simulink model "RL_RefAdjSup"  (R2025b)
settings: Solver=ode14x  StartTime=0.0  StopTime=10.0  FixedStep=Ts_local  RelTol=1e-3
model workspace (MAT data in the model file):
  FSI_max = [111.58614649; 109.244229433; 111.951462771]
  FSI_min = [3.65502707696; 3.64264743495; 3.42913459589]
  K1 = 1
  K2 = 1e-06
  Ncycle = 25
  SampEn_max = [0.399850516102; 0.373441099122; 0.45958437331]
  SampEn_min = [0.118794892672; 0.117721768048; 0.119599512992]
  fs = 5000
  m = 2
  rRatio = 0.2
values from neighbouring files (symbols this model uses):
  f = 50.0    [ctrlSys.sldd]
  Ts_ctrl = 0.1    [ctrlSys.sldd]
  Ts_local = 1.0E-5    [ctrlSys.sldd]
  Ts_meas = 0.005    [ctrlSys.sldd]
libraries: rllib x1
settings Model: DataDictionary=ctrlSys.sldd  Creator=i336  LastModifiedBy=LYG

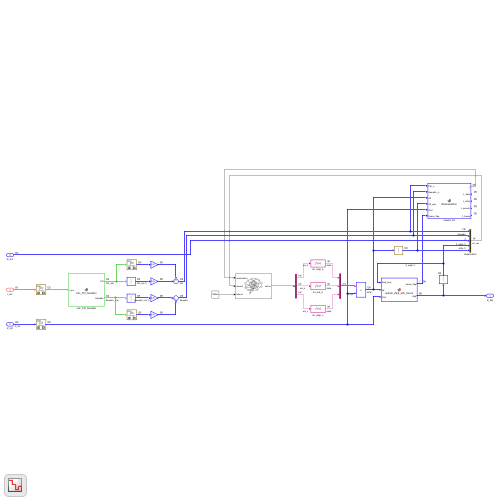
[thumbnail: Simulink's stored preview of the top-level diagram]
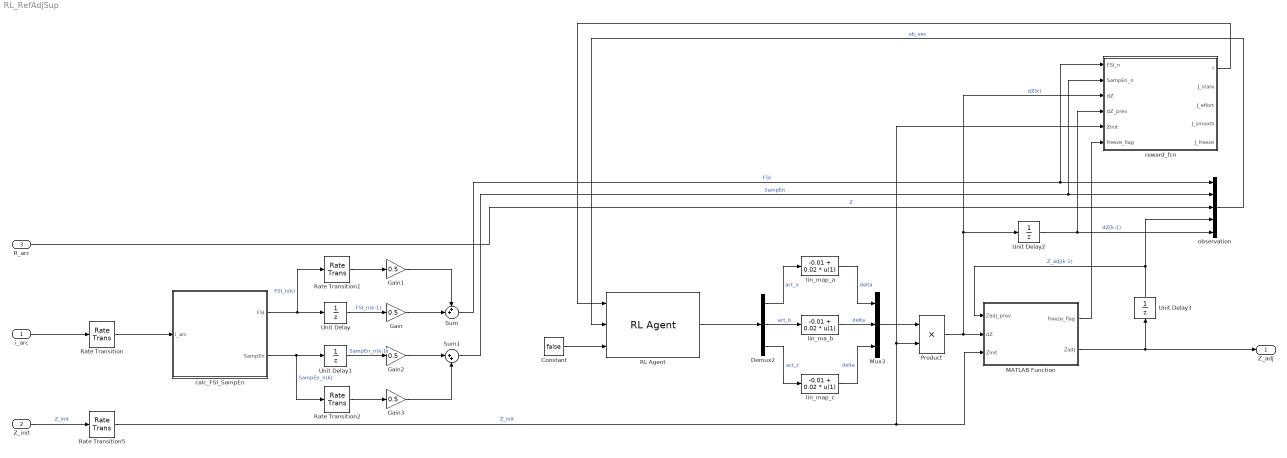
== system RL_RefAdjSup ==
  i_arc : Inport  SampleTime=Ts_local
  Z_init : Inport  Port=2  PortDimensions=[3 1]  SampleTime=Ts_ctrl
  R_arc : Inport  Port=3  PortDimensions=3  SampleTime=Ts_meas
  Constant : Constant  Value=false
  Demux2 : Demux  Outputs=3
  Gain{,1..3} (4 alike) : Gain  Gain=0.5
  MATLAB Function : MATLAB Function  TreatAsAtomicUnit=on
  Mux3 : Mux  Inputs=3
  Product : Product
  RL Agent : rllib/RL Agent  Agent=agentObj  ExternalActionAsInput=off  ProvideLastAction=off  ProvideCumRwd=off  TreatAsDirectFeedthrough=on  UseStrictObservationDataTypes=off
  Rate Transition : RateTransition  OutPortSampleTime=1 / fs
  Rate Transition1 : RateTransition  OutPortSampleTime=Ncycle * (1 / f)
  Rate Transition2 : RateTransition  OutPortSampleTime=Ncycle * (1 / f)
  Rate Transition5 : RateTransition  OutPortSampleTime=Ts_sup
  Sum : Sum  Inputs=++|
  Sum1 : Sum  Inputs=|++
  Unit Delay : UnitDelay  SampleTime=Ncycle * (1 / f)  HasFrameUpgradeWarning=on
  Unit Delay1 : UnitDelay  SampleTime=Ncycle * (1 / f)  HasFrameUpgradeWarning=on
  Unit Delay2 : UnitDelay  SampleTime=-1  HasFrameUpgradeWarning=on
  Unit Delay3 : UnitDelay  SampleTime=-1  HasFrameUpgradeWarning=on
  calc_FSI_SampEn : MATLAB Function  TreatAsAtomicUnit=on  SystemSampleTime=1 / fs
  lin_ma_b : Fcn  Expr=-0.01 + 0.02 * u(1)
  lin_map_a : Fcn  Expr=-0.01 + 0.02 * u(1)
  lin_map_c : Fcn  Expr=-0.01 + 0.02 * u(1)
  observation : Mux  Inputs=5
  reward_fcn : MATLAB Function  TreatAsAtomicUnit=on
  Z_adj : Outport
  wires:
  i_arc/1 -> Rate Transition/1
  Rate Transition/1 -> calc_FSI_SampEn/1(i_arc)
  calc_FSI_SampEn/1(FSI) -> Rate Transition1/1, Unit Delay/1  "FSI_n(k)"
  calc_FSI_SampEn/2(SampEn) -> Rate Transition2/1, Unit Delay1/1  "SampEn_n(k)"
  Unit Delay/1 -> Gain/1  "FSI_n(k-1)"
  Gain/1 -> Sum/2
  Gain1/1 -> Sum/1
  Gain2/1 -> Sum1/1
  Gain3/1 -> Sum1/2
  Unit Delay1/1 -> Gain2/1  "SampEn_n(k-1)"
  Rate Transition1/1 -> Gain1/1
  Rate Transition2/1 -> Gain3/1
  Z_init/1 -> Rate Transition5/1  "Z_init"
  Mux3/1 -> Product/1
  lin_map_a/1 -> Mux3/1  "delta"
  lin_ma_b/1 -> Mux3/2  "delta"
  lin_map_c/1 -> Mux3/3  "delta"
  Sum/1 -> reward_fcn/1(FSI_n), observation/1  "FSI"
  Sum1/1 -> reward_fcn/2(SampEn_n), observation/2  "SampEn"
  Rate Transition5/1 -> MATLAB Function/3(Zinit), Product/2, reward_fcn/5(Zinit)  "Z_init"
  Product/1 -> MATLAB Function/2(dZ), reward_fcn/3(dZ), Unit Delay2/1  "dZ(k)"
  MATLAB Function/2(Zadj) -> Z_adj/1, Unit Delay3/1
  Unit Delay3/1 -> observation/4, MATLAB Function/1(Zadj_prev)  "Z_adj(k-1)"
  R_arc/1 -> observation/3  "Z"
  Unit Delay2/1 -> reward_fcn/4(dZ_prev), observation/5  "dZ(k-1)"
  MATLAB Function/1(freeze_flag) -> reward_fcn/6(freeze_flag)
  Demux2/1 -> lin_map_a/1  "act_a"
  Demux2/2 -> lin_ma_b/1  "act_b"
  Demux2/3 -> lin_map_c/1  "act_c"
  Constant/1 -> RL Agent/3
  RL Agent/1 -> Demux2/1
  observation/1 -> RL Agent/2  "ob_vec"
  reward_fcn/1(r) -> RL Agent/1

== matlab function RL_RefAdjSup/reward_fcn ==
  data: FSI_n input; r output; SampEn_n input; dZ input; dZ_prev input; Zinit input; freeze_flag input; J_state output; J_effort output; J_smooth output; J_freeze output
function [r, J_state, J_effort, J_smooth, J_freeze] = RLRewardFcn( ...
    FSI_n, SampEn_n, dZ, dZ_prev, Zinit, freeze_flag)
%#codegen
% RL reward for variable-impedance supervisory control
%
% Inputs:
%   FSI_n       : 3x1 normalized FSI in [0,1]
%   SampEn_n    : 3x1 normalized SampEn in [0,1]
%   dZ          : 3x1 current impedance increment (physical value)
%   dZ_prev     : 3x1 previous impedance increment (physical value)
%   Zinit       : 3x1 initial/base impedance
%   freeze_flag : 3x1, 1 if corresponding phase update is frozen, else 0
%
% Outputs:
%   r           : scalar reward
%   J_state     : state-quality cost
%   J_effort    : control-effort cost
%   J_smooth    : smoothness cost
%   J_freeze    : freeze penalty cost

    % ---------- Hard-coded weights ----------
    alphaF = 1.0;   % weight of FSI term inside state cost
    alphaS = 1.0;   % weight of SampEn term inside state cost

    beta1  = 0.10;  % weight of effort penalty
    beta2  = 0.20;  % weight of smoothness penalty
    beta3  = 0.50;  % weight of freeze penalty
    % ----------------------------------------

    % Ensure column vectors
    FSI_n       = FSI_n(:);
    SampEn_n    = SampEn_n(:);
    dZ          = dZ(:);
    dZ_prev     = dZ_prev(:);
    Zinit       = Zinit(:);
    freeze_flag = freeze_flag(:);

    % Clamp normalized features to [0,1] for safety
    FSI_n    = min(max(FSI_n, 0.0), 1.0);
    SampEn_n = min(max(SampEn_n, 0.0), 1.0);

    % Convert physical dZ to normalized action-like variable in [-1,1]
    %
    % Forward mapping used previously:
    %   dZ = Zinit * (-0.01 + 0.02 * a),   a in [-1,1]
    %
    % Inverse mapping:
    %   a = (dZ./Zinit + 0.01) / 0.02
    %
    % This normalization makes the effort/smoothness terms dimensionless.
    eps_z = 1e-9;
    Zsafe = max(abs(Zinit), eps_z);

    dZ_n      = (dZ      ./ Zsafe + 0.01) / 0.02;
    dZ_prev_n = (dZ_prev ./ Zsafe + 0.01) / 0.02;

    % Optional clamping for robustness
    dZ_n      = min(max(dZ_n,      -1.0), 1.0);
    dZ_prev_n = min(max(dZ_prev_n, -1.0), 1.0);

    % 1) Buried-arc state cost
    % Larger FSI is better, smaller SampEn is better
    J_state = sum(alphaF * (1.0 - FSI_n) + alphaS * SampEn_n);

    % 2) Control-effort cost
    J_effort = sum(dZ_n.^2);

    % 3) Smoothness cost
    J_smooth = sum((dZ_n - dZ_prev_n).^2);

    % 4) Freeze penalty
    J_freeze = sum(freeze_flag ~= 0);

    % Final reward
    r = -J_state ...
        - beta1 * J_effort ...
        - beta2 * J_smooth ...
        - beta3 * J_freeze;
end

== matlab function RL_RefAdjSup/calc_FSI_SampEn ==
  data: i_arc input size=[3 1]; FSI output; SampEn output; K1 parameter size=[1 1]; K2 parameter size=[1 1]; fs parameter size=[1 1]; Ncycle parameter size=[1 1]; f parameter size=[1 1]; m parameter size=[1 1]; rRatio parameter size=[1 1]; FSI_max parameter size=[3 1]; FSI_min parameter size=[3 1]; SampEn_max parameter size=[3 1]; SampEn_min parameter size=[3 1]
function [FSI, SampEn] = calc_FSI_SampEn( ...
    i_arc, K1, K2, fs, Ncycle, f, m, rRatio, ...
    FSI_max, FSI_min, SampEn_max, SampEn_min)
%#codegen
% i_arc   : 3x1 instantaneous arc current [ia; ib; ic]
% FSI     : 3x1 normalized FSI of three phases
% SampEn  : 3x1 normalized sample entropy of three phases
%
% This version:
% 1) stores samples every call,
% 2) computes features only once every Nhop samples,
% 3) holds the last computed outputs between updates.

    Nwin = int32(Ncycle * fs / f);   % assume exact integer
    Nhop = Nwin;                     % non-overlapping windows
    % For overlapped windows, e.g.:
    % Nhop = int32(Nwin/2);

    persistent buf head count sinceCalc lastFSI lastSampEn

    if isempty(head)
        buf        = zeros(Nwin, 3);
        head       = int32(0);
        count      = int32(0);
        sinceCalc  = int32(0);
        lastFSI    = zeros(3,1);
        lastSampEn = zeros(3,1);
    end

    % Ensure column vector
    i_arc = reshape(i_arc, 3, 1);

    % -------------------------
    % 1) Update circular buffer
    % -------------------------
    head = head + 1;
    if head > Nwin
        head = int32(1);
    end

    buf(head, :) = i_arc.';

    if count < Nwin
        count = count + 1;
    end

    sinceCalc = sinceCalc + 1;

    % Default outputs: hold last values
    FSI    = lastFSI;
    SampEn = lastSampEn;

    % Before first full window, output zeros
    if count < Nwin
        FSI(:)    = 0.0;
        SampEn(:) = 0.0;
        return;
    end

    % -----------------------------------------
    % 2) Only recompute once every Nhop samples
    % -----------------------------------------
    if sinceCalc < Nhop
        return;
    end
    sinceCalc = int32(0);

    % Reconstruct ordered window: oldest --> newest
    xwin = zeros(Nwin, 3);
    if head < Nwin
        n1 = Nwin - head;
        xwin(1:n1, :)      = buf(head+1:Nwin, :);
        xwin(n1+1:Nwin, :) = buf(1:head, :);
    else
        xwin = buf;
    end

    % Compute features phase by phase
    for p = 1:3
        x = xwin(:, p);

        fsi_raw = local_fsi(x, fs, f, K1, K2);
        den1 = FSI_max(p) - FSI_min(p);
        if abs(den1) <= 1e-12
            FSI(p) = 0.0;
        else
            FSI_n = (fsi_raw - FSI_min(p)) / den1;
            FSI(p) = min(max(FSI_n, 0.0), 1.0);
        end

        se_raw = local_sampen(x, m, rRatio);
        den2 = SampEn_max(p) - SampEn_min(p);
        if abs(den2) <= 1e-12
            SampEn(p) = 0.0;
        else
            SampEn_n = (se_raw - SampEn_min(p)) / den2;
            SampEn(p) = min(max(SampEn_n, 0.0), 1.0);
        end
    end

    % Save outputs for holding until next update
    lastFSI    = FSI;
    lastSampEn = SampEn;
end

function y = local_fsi(x, fs, f0, K1, K2)
% Compute FSI from one phase current window

    x = x(:);
    N = length(x);

    % Remove DC component
    x = x - mean(x);

    % FFT
    X = fft(x);

    % Single-sided amplitude spectrum
    nHalf = floor(N/2) + 1;
    A = 2.0 * abs(X(1:nHalf)) / N;
    A(1) = abs(X(1)) / N;
    if mod(N, 2) == 0
        A(end) = abs(X(nHalf)) / N;
    end

    % Extract harmonic amplitudes H1 ... H20
    H = zeros(20, 1);
    for h = 1:20
        k = round(h * f0 / fs * N) + 1;
        if k >= 1 && k <= nHalf
            H(h) = A(k);
        else
            H(h) = 0.0;
        end
    end

    denom = K1 * sqrt(sum(H(10:20).^2)) + K2;

    if denom <= 1e-12
        y = 0.0;
    else
        y = H(1) / denom;
    end
end

function se = local_sampen(x, m, rRatio)
% Compute sample entropy of one phase current window

    x = x(:);
    N = length(x);

    if N <= m + 1
        se = 0.0;
        return;
    end

    sigma = std(x);
    r = rRatio * sigma;

    if r <= 1e-12
        se = 0.0;
        return;
    end

    A = 0.0;
    B = 0.0;

    Nm = N - m;

    for i = 1:Nm
        for j = i+1:Nm
            match_m = true;

            for k = 0:m-1
                if abs(x(i+k) - x(j+k)) > r
                    match_m = false;
                    break;
                end
            end

            if match_m
                B = B + 1.0;

                if abs(x(i+m) - x(j+m)) <= r
                    A = A + 1.0;
                end
            end
        end
    end

    se = -log((A + realmin) / (B + realmin));
end

== matlab function RL_RefAdjSup/MATLAB Function ==
  data: freeze_flag output; Zadj_prev input; Zadj output; dZ input; Zinit input
function [freeze_flag, Zadj] = update_Zadj_with_freeze(Zadj_prev, dZ, Zinit)
%#codegen
% Zadj_prev, dZ, Zinit: 3x1 vectors
% Zadj: updated 3x1 vector
% freeze_flag: 3x1 logical/double vector

    Zadj_prev = Zadj_prev(:);
    dZ        = dZ(:);
    Zinit     = Zinit(:);

    Zcand = Zadj_prev + dZ;
    lower = -0.1 .* Zinit;
    upper = zeros(3,1);

    freeze_flag = (Zcand > upper) | (Zcand < lower);

    Zadj = Zcand;
    Zadj(freeze_flag) = Zadj_prev(freeze_flag);
end
